simulink model "simTanque"  (R2020b)
settings: Solver=VariableStepAuto  StartTime=0.0  StopTime=500  RelTol=1e-3
values from neighbouring files (symbols this model uses):
  A = pi    (= 3.14159265359)    [ControlNivel.m]
  h0 = 1.5    [ControlNivel.m]
  Ke = 0.25/10    (= 0.025)    [ControlNivel.m]
  Ks = 0.3543/(10*sqrt(3))    [ControlNivel.m]
  u20 = 5.0    (= 5)    [ControlNivel.m]
libraries: pid_lib x1
settings Model: Creator=serbogr1  LastModifiedBy=bou

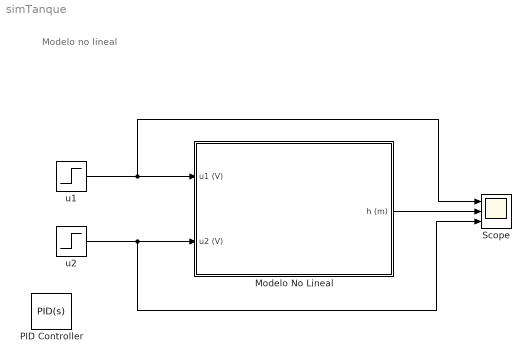
== system simTanque ==
  note: Modelo no lineal
  Modelo No Lineal : Subsystem
  PID Controller : pid_lib/PID Controller  Controller=PID  Form=Parallel  TimeDomain=Continuous-time  UseExternalTs=off  SampleTime=-1  IntegratorMethod=Forward Euler  FilterMethod=Forward Euler  ControllerParametersSource=internal  P=1  I=1  D=0  UseFilter=on  N=100  TunerSelectOption=Transfer Function Based (PID Tuner App)  InitialConditionSource=internal  InitialConditionForIntegrator=0  InitialConditionForFilter=0  DifferentiatorICPrevScaledInput=0  ExternalReset=none  TrackingMode=off  Kt=1  LimitOutput=off  SatLimitsSource=internal  UpperSaturationLimit=inf  LowerSaturationLimit=-inf  LinearizeAsGain=on  AntiWindupMode=none  Kb=1  POutMin=[]  POutMax=[]  IOutMin=[]  IOutMax=[]  DOutMin=[]  DOutMax=[]  NOutMin=[]  NOutMax=[]  SumOutMin=[]  SumOutMax=[]  SaturationOutMin=[]  SaturationOutMax=[]  PParamMin=[]  PParamMax=[]  IParamMin=[]  IParamMax=[]  DParamMin=[]  DParamMax=[]  NParamMin=[]  NParamMax=[]  KbParamMin=[]  KbParamMax=[]  KtParamMin=[]  KtParamMax=[]  KbOutMin=[]  KbOutMax=[]  KtOutMin=[]  KtOutMax=[]  IntegratorOutMin=[]  IntegratorOutMax=[]  FilterOutMin=[]  FilterOutMax=[]  SumI1OutMin=[]  SumI1OutMax=[]  SumI2OutMin=[]  SumI2OutMax=[]  SumI3OutMin=[]  SumI3OutMax=[]  SumI4OutMin=[]  SumI4OutMax=[]  SumDOutMin=[]  SumDOutMax=[]  DifferentiatorOutMin=[]  DifferentiatorOutMax=[]  FilterDiffOutCoefMin=[]  FilterDiffOutCoefMax=[]  ReciprocalOutMin=[]  ReciprocalOutMax=[]  SumDenOutMin=[]  SumDenOutMax=[]  SumNumOutMin=[]  SumNumOutMax=[]  DivideOutMin=[]  DivideOutMax=[]  UdiffTsProdOutMin=[]  UdiffTsProdOutMax=[]  NTsProdOutMin=[]  NTsProdOutMax=[]  UintegralTsProdOutMin=[]  UintegralTsProdOutMax=[]  UngainTsProdOutMin=[]  UngainTsProdOutMax=[]  IntegratorContinuousStateAttributes=''  IntegratorStateMustResolveToSignalObject=off  IntegratorRTWStateStorageClass=Auto  FilterContinuousStateAttributes=''  FilterStateMustResolveToSignalObject=off  FilterRTWStateStorageClass=Auto  ParallelPVariant=InternalParameters  IdealPVariant=Disabled  IVariant=InternalParameters  DVariant=InternalParameters  IntegratorVariant=Continuous  SatVariant=Disabled  AWVariant=Passthrough  PCopyVariant=Disabled  TRVariant=Disabled  FdbkBlocksVariant=Forward  IdealPFdbkVariant=Disabled  SatFdbkVariant=Disabled  DerivativeFilterVariant=ContFilter  NVariant=InternalParameters  NCopyVariant=Disabled  FilterICVariant=InternalICsFilter  IntegratorICVariant=InternalICs  ExternalResetVariant=Disabled  TRSumVariant=Passthrough  SumFdbkVariant=Disabled  SumVariant=Sum_PID  TsampFilterVariant=InternalTs  TsampNgainVariant=Passthrough  TsampIntegralVariant=Passthrough  ExternalSaturationOutDataTypeStr=Inherit: Same as second input
  Scope : Scope  NumInputPorts=3
  "u1 " : Step  Before=Ke*u20/(Ks*sqrt(h0))  After=Ke*u20/(Ks*sqrt(h0))  SampleTime=0
  "u2 " : Step  Before=5.0  After=5.0  SampleTime=0
  wires:
  "u2 "/1 -> Modelo No Lineal/2(u2 (V)), Scope/3
  "u1 "/1 -> Scope/1, Modelo No Lineal/1(u1 (V))
  Modelo No Lineal/1(h (m)) -> Scope/2

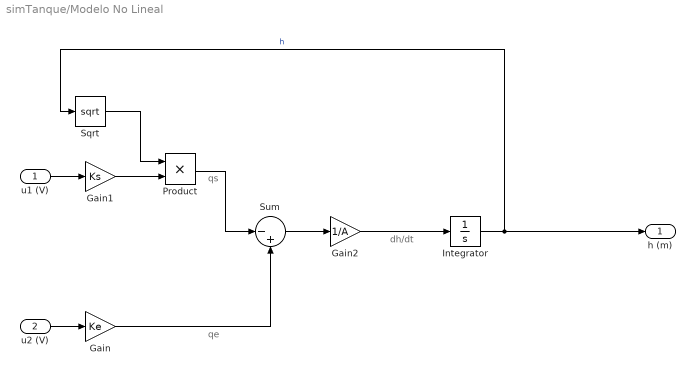
== system simTanque/Modelo No Lineal ==
  note: qe
  note: qs
  note: dh/dt
  u1 (V) : Inport
  u2 (V) : Inport  Port=2
  Gain : Gain  Gain=Ke
  Gain1 : Gain  Gain=Ks
  Gain2 : Gain  Gain=1/A
  Integrator : Integrator  InitialCondition=h0
  Product : Product
  Sqrt : Sqrt  SaturateOnIntegerOverflow=on
  Sum : Sum  Inputs=|-+
  h (m) : Outport
  wires:
  Integrator/1 -> h (m)/1, Sqrt/1  "h"
  Gain/1 -> Sum/2
  Gain2/1 -> Integrator/1
  Sqrt/1 -> Product/1
  Sum/1 -> Gain2/1
  u1 (V)/1 -> Gain1/1
  u2 (V)/1 -> Gain/1
  Product/1 -> Sum/1
  Gain1/1 -> Product/2
